simulink model "Example_MotionFilter3DoF"  (R2025a)
settings: Solver=FixedStepAuto  StartTime=0.0  StopTime=180  FixedStep=0.01  RelTol=1e-3  EnableMultiTasking=on
values from neighbouring files (symbols this model uses):
  model_matB = [0.000237948834266 -0.000004551592718 0.000010003488944; -0.000009313932115 0.000215194147058 -0.000024957572224; -0.000002202124158 -0.000002930260852 0.000043018345190]    [INIT.m]
  model_matF = [-0.031604977390302 0 0 0.233741474945168 0 0 0.133462292221887 -0.020792892088185 0 0; 0 -0.041708610292712 0.017242263124379 0 -0.251243228165994 -0.000476044356140 0.005297185500344 0 -0.167981638498434 0.497442136687157; 0 0.000017966020615 -0.023528504195578 0 0.000108223241795 0.000649602175186 -0.000002281767319 0 0.000072358238719 -0.678801229030825]    [INIT.m]
  model_stddev_externalXYN = [10; 10; 3] * 1e-3    [INIT.m]
  model_stddev_velocityUVR = [10; 10; 1] * 1e-5    [INIT.m]
undefined symbols (not defined in the file or in its folder): input, measurement, model, reset, stddevMeasurement, stddevModel, structMotionFilter3DoFIn
libraries: simulink_extras x4, AVE_Library x2, MotionFilter_Library x1
settings Model: Creator=damerius  LastModifiedBy=damerius
settings SolverCC: ConcurrentTasks=on
settings DataIOCC: SaveOutput=off  SignalLogging=off  DSMLogging=off  SaveTime=off  ReturnWorkspaceOutputs=off
settings OptimizationCC: DefaultParameterBehavior=Inlined  ZeroExternalMemoryAtStartup=off  ZeroInternalMemoryAtStartup=off  SimCompilerOptimization=on
settings DebuggingCC: UnconnectedInputMsg=warning  UnconnectedOutputMsg=warning  UnconnectedLineMsg=warning
settings HardwareCC: ProdBitPerLong=64.0  ProdHWDeviceType=Intel->x86-64 (Linux 64)  TargetBitPerLong=64.0  TargetBitPerPointer=64.0  TargetBitPerSizeT=64.0  TargetBitPerPtrDiffT=64.0  TargetLargestAtomicFloat=Float  TargetIntDivRoundTo=Zero  TargetEndianess=LittleEndian  TargetWordSize=64.0  TargetHWDeviceType=Intel->x86-64 (Linux 64)  ProdEqTarget=off
settings ModelReferenceCC: EnableRefExpFcnMdlSchedulingChecks=on
settings SFSimCC: SimParseCustomCode=off  SimGenImportedTypeDefs=on  SimTargetLang=C++  SimDLTargetLibrary=mkl-dnn
settings RTWCC: GenCodeOnly=on  PackageGeneratedCodeAndArtifacts=on  PackageName=PackNGo  BuildConfiguration=Faster Runs  TargetLang=C++
settings CodeAppCC: ForceParamTrailComments=on  MaxIdLength=128.0  StateflowObjectComments=on  MATLABSourceComments=on  UseSimReservedNames=on
settings GRTTargetCC: TargetLangStandard=C++11 (ISO)  MatFileLogging=off  CodeInterfacePackaging=C++ class  SubcomponentCodeInterfacePackaging=C++ class

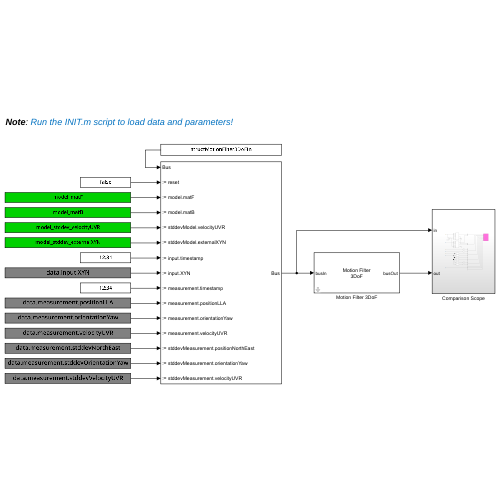
[thumbnail: Simulink's stored preview of the top-level diagram]
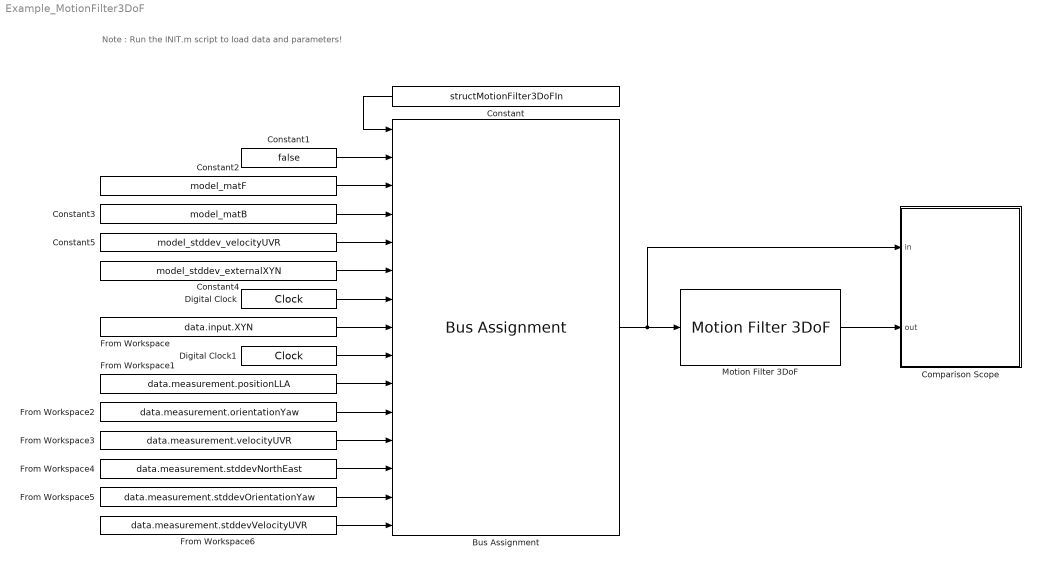
== system Example_MotionFilter3DoF ==
  note: Note : Run the INIT.m script to load data and parameters!
  Bus Assignment : BusAssignment  AssignedSignals=reset,model.matF,model.matB,stddevModel.velocityUVR,stddevModel.externalXYN,input.timestamp,input.XYN,measurement.timestamp,measurement.positionLLA,measurement.orientationYaw,measurement.velocityUVR,stddevMeasurement.positionNorthEast,stddevMeasurement.orientationYaw,stddevMeasurement.velocityUVR
  Comparison Scope : Subsystem
  Constant : Constant  Value=structMotionFilter3DoFIn  OutDataTypeStr=Bus: busMotionFilter3DoFIn
  Constant1 : Constant  Value=false  OutDataTypeStr=boolean
  Constant2 : Constant  Value=model_matF
  Constant3 : Constant  Value=model_matB
  Constant4 : Constant  Value=model_stddev_externalXYN
  Constant5 : Constant  Value=model_stddev_velocityUVR
  Digital Clock : DigitalClock  SampleTime=0.01
  Digital Clock1 : DigitalClock  SampleTime=0.01
  From Workspace : FromWorkspace  VariableName=data.input.XYN  SampleTime=0.01  Interpolate=off  OutputAfterFinalValue=Holding final value
  From Workspace1 : FromWorkspace  VariableName=data.measurement.positionLLA  SampleTime=0.01  Interpolate=off  OutputAfterFinalValue=Holding final value
  From Workspace2 : FromWorkspace  VariableName=data.measurement.orientationYaw  SampleTime=0.01  Interpolate=off  OutputAfterFinalValue=Holding final value
  From Workspace3 : FromWorkspace  VariableName=data.measurement.velocityUVR  SampleTime=0.01  Interpolate=off  OutputAfterFinalValue=Holding final value
  From Workspace4 : FromWorkspace  VariableName=data.measurement.stddevNorthEast  SampleTime=0.01  Interpolate=off  OutputAfterFinalValue=Holding final value
  From Workspace5 : FromWorkspace  VariableName=data.measurement.stddevOrientationYaw  SampleTime=0.01  Interpolate=off  OutputAfterFinalValue=Holding final value
  From Workspace6 : FromWorkspace  VariableName=data.measurement.stddevVelocityUVR  SampleTime=0.01  Interpolate=off  OutputAfterFinalValue=Holding final value
  Motion Filter 3DoF : MotionFilter_Library/Motion Filter 3DoF
  wires:
  Constant/1 -> Bus Assignment/1
  Bus Assignment/1 -> Comparison Scope/1(in), Motion Filter 3DoF/1
  Constant1/1 -> Bus Assignment/2
  Constant2/1 -> Bus Assignment/3
  Constant3/1 -> Bus Assignment/4
  From Workspace/1 -> Bus Assignment/8
  From Workspace1/1 -> Bus Assignment/10
  From Workspace2/1 -> Bus Assignment/11
  From Workspace3/1 -> Bus Assignment/12
  From Workspace4/1 -> Bus Assignment/13
  From Workspace5/1 -> Bus Assignment/14
  From Workspace6/1 -> Bus Assignment/15
  Digital Clock/1 -> Bus Assignment/7
  Digital Clock1/1 -> Bus Assignment/9
  Constant5/1 -> Bus Assignment/5
  Constant4/1 -> Bus Assignment/6
  Motion Filter 3DoF/1 -> Comparison Scope/2(out)

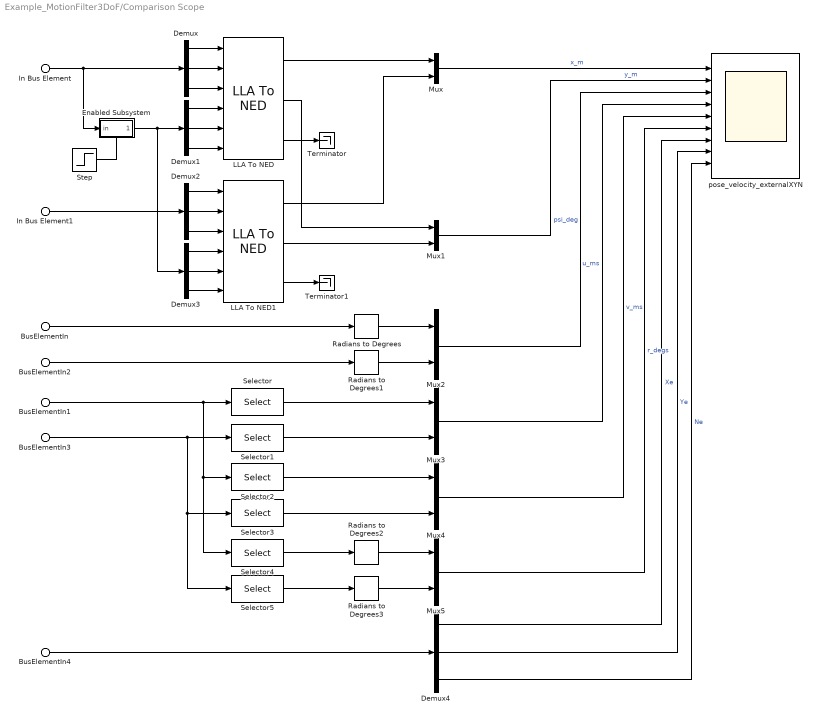
== system Example_MotionFilter3DoF/Comparison Scope ==
  In Bus Element : Inport  PortName=in  Element=measurement.positionLLA
  BusElementIn : Inport  PortName=in  Element=measurement.orientationYaw
  BusElementIn1 : Inport  PortName=in  Element=measurement.velocityUVR
  In Bus Element1 : Inport  Port=2  PortName=out  Element=motion.positionLLA
  BusElementIn2 : Inport  Port=2  PortName=out  Element=motion.orientationYaw
  BusElementIn3 : Inport  Port=2  PortName=out  Element=motion.velocityUVR
  BusElementIn4 : Inport  Port=2  PortName=out  Element=disturbance.XYN
  Demux{,1..4} (5 alike) : Demux  Outputs=3
  Enabled Subsystem : Subsystem  TreatAsAtomicUnit=on
  LLA To NED : AVE_Library/Essential/Transformation/LLA To NED
      settings: SourceProductName=AVE - Autonomous Vehicle Control Toolbox
  LLA To NED1 : AVE_Library/Essential/Transformation/LLA To NED
      settings: SourceProductName=AVE - Autonomous Vehicle Control Toolbox
  Mux{,1..5} (6 alike) : Mux  Inputs=2
  Radians to Degrees{,1..3} (4 alike) : simulink_extras/Transformations/Radians to Degrees
  Selector : Selector  InputPortWidth=3  IndexOptions=Index vector (dialog)  Indices=1  OutputSizes=1
  Selector1 : Selector  InputPortWidth=3  IndexOptions=Index vector (dialog)  Indices=1  OutputSizes=1
  Selector2 : Selector  InputPortWidth=3  IndexOptions=Index vector (dialog)  Indices=2  OutputSizes=1
  Selector3 : Selector  InputPortWidth=3  IndexOptions=Index vector (dialog)  Indices=2  OutputSizes=1
  Selector4 : Selector  InputPortWidth=3  IndexOptions=Index vector (dialog)  Indices=3  OutputSizes=1
  Selector5 : Selector  InputPortWidth=3  IndexOptions=Index vector (dialog)  Indices=3  OutputSizes=1
  Step : Step  Time=0.01  Before=1  After=0  SampleTime=0.01
  Terminator : Terminator
  Terminator1 : Terminator
  pose_velocity_externalXYN : Scope  NumInputPorts=9
      settings: ActiveDisplayYMinimum=-44.508029688328435  ActiveDisplayYMaximum=5.2284363744473143
  wires:
  Demux/3 -> LLA To NED/3
  Demux/2 -> LLA To NED/2
  Demux/1 -> LLA To NED/1
  In Bus Element/1 -> Enabled Subsystem/1(in), Demux/1
  Enabled Subsystem/1(Out1) -> Demux1/1, Demux3/1
  Step/1 -> Enabled Subsystem/Enable
  Demux2/1 -> LLA To NED1/1
  Demux2/2 -> LLA To NED1/2
  Demux2/3 -> LLA To NED1/3
  In Bus Element1/1 -> Demux2/1
  Demux1/1 -> LLA To NED/4
  Demux1/2 -> LLA To NED/5
  Demux1/3 -> LLA To NED/6
  Demux3/1 -> LLA To NED1/4
  Demux3/2 -> LLA To NED1/5
  Demux3/3 -> LLA To NED1/6
  LLA To NED/3 -> Terminator/1
  LLA To NED1/3 -> Terminator1/1
  LLA To NED/1 -> Mux/1
  LLA To NED1/1 -> Mux/2
  LLA To NED/2 -> Mux1/1
  LLA To NED1/2 -> Mux1/2
  Radians to Degrees/1 -> Mux2/1
  Radians to Degrees1/1 -> Mux2/2
  BusElementIn/1 -> Radians to Degrees/1
  BusElementIn2/1 -> Radians to Degrees1/1
  Mux/1 -> pose_velocity_externalXYN/1  "x_m"
  Mux1/1 -> pose_velocity_externalXYN/2  "y_m"
  Mux2/1 -> pose_velocity_externalXYN/3  "psi_deg"
  BusElementIn1/1 -> Selector4/1, Selector2/1, Selector/1
  BusElementIn3/1 -> Selector5/1, Selector3/1, Selector1/1
  Selector/1 -> Mux3/1
  Selector1/1 -> Mux3/2
  Selector3/1 -> Mux4/2
  Selector2/1 -> Mux4/1
  Selector4/1 -> Radians to Degrees2/1
  Selector5/1 -> Radians to Degrees3/1
  Radians to Degrees2/1 -> Mux5/1
  Radians to Degrees3/1 -> Mux5/2
  Mux3/1 -> pose_velocity_externalXYN/4  "u_ms"
  Mux4/1 -> pose_velocity_externalXYN/5  "v_ms"
  Mux5/1 -> pose_velocity_externalXYN/6  "r_degs"
  BusElementIn4/1 -> Demux4/1
  Demux4/1 -> pose_velocity_externalXYN/7  "Xe"
  Demux4/2 -> pose_velocity_externalXYN/8  "Ye"
  Demux4/3 -> pose_velocity_externalXYN/9  "Ne"

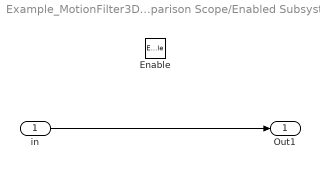
== system Example_MotionFilter3DoF/Comparison Scope/Enabled Subsystem ==
  in : Inport
  Enable : EnablePort
  Out1 : Outport
  wires:
  in/1 -> Out1/1
